simulink model "new_fusion_model"  (R2026a)
settings: Solver=VariableStepAuto  StopTime=180
InitFcn:
  | initNoise
  | initUKF
  | initKF
model workspace (MAT data in the model file):
  Ts = 0.05
undefined symbols (not defined in the file): Discrete, r_range, r_th_ac, r_th_ir, r_th_radar, Rkf, seed_ac, seed_ir, seed_radar_bearing, seed_radar_range, Time, x0kf
libraries: sharedTrackingLibrary x3, ctrlSharedLib x1

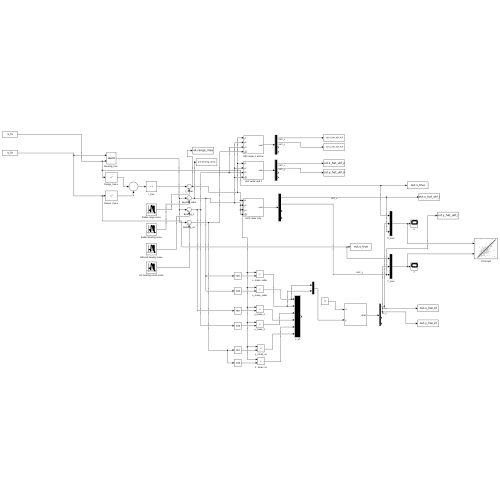
[thumbnail: Simulink's stored preview of the top-level diagram]
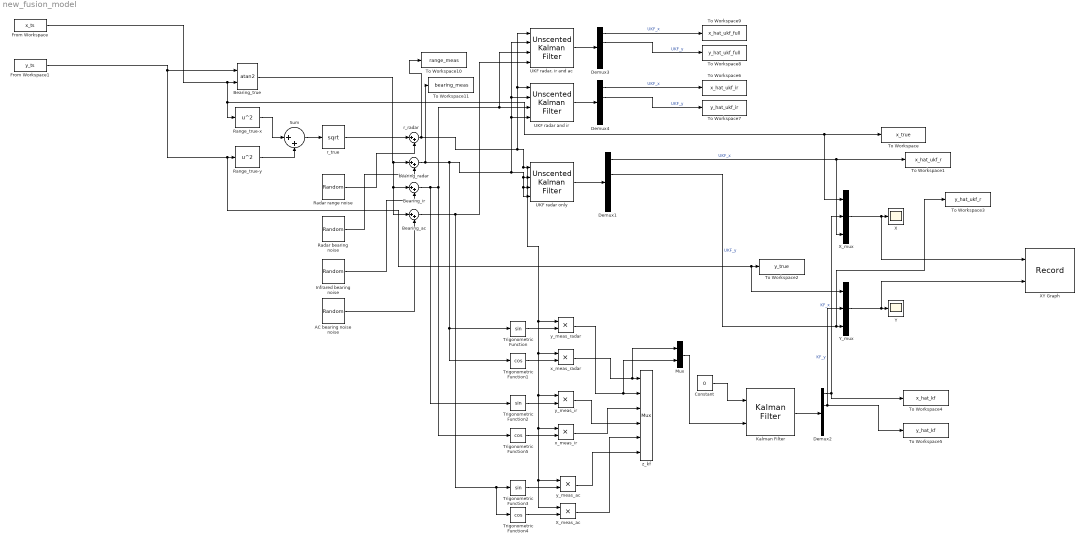
== system new_fusion_model ==
  AC bearing noise noise : RandomNumber  Variance=r_th_ac  Seed=seed_ac  SampleTime=4*Ts
  Bearing_ac : Sum  Inputs=|++
  Bearing_ir : Sum  Inputs=|++
  "Bearing_true " : Trigonometry  Operator=atan2
  Constant : Constant  Value=0
  Demux{1..4} (4 alike) : Demux
  From Workspace : FromWorkspace  VariableName=x_ts  SampleTime=Ts
  From Workspace1 : FromWorkspace  VariableName=y_ts  SampleTime=Ts
  Infrared bearing noise : RandomNumber  Variance=r_th_ir  Seed=seed_ir  SampleTime=2*Ts
  Kalman Filter : ctrlSharedLib/Kalman Filter  TimeDomain=Discrete-Time  UseCurrentEstimator=on  ModelSource=LTI State-Space Variable  ModelSourceVariable=sysKF  A=0.95  B=1  C=1  D=0  NumberOfStates=1  NumberOfInputs=1  NumberOfOutputs=1  Ts=-1  InitialEstimateSource=Dialog  X0=x0kf  P0=10  UseK=off  UseGH=off  G=1  TimeInvariantG=on  H=0  TimeInvariantH=on  NumberOfProcessNoiseInputs=1  Q=Qkf  TimeInvariantQ=on  R=Rkf  TimeInvariantR=on  N=0  TimeInvariantN=on  AddInputPort=on  AddEnablePort=off  OutputEstimatedY=off  OutputP=off
  Mux : Mux  Inputs=2
  Radar bearing noise : RandomNumber  Variance=r_th_radar  Seed=seed_radar_bearing  SampleTime=Ts
  Radar range noise : RandomNumber  Variance=r_range  Seed=seed_radar_range  SampleTime=Ts
  Range_true-x : Math  Operator=square
  Range_true-y : Math  Operator=square
  Sum : Sum  Inputs=|++
  To Workspace : ToWorkspace  VariableName=x_true  SaveFormat=Timeseries  SampleTime=Ts
  To Workspace1 : ToWorkspace  VariableName=x_hat_ukf_r  SaveFormat=Timeseries  SampleTime=Ts
  To Workspace10 : ToWorkspace  VariableName=range_meas  SaveFormat=Timeseries  SampleTime=Ts
  To Workspace11 : ToWorkspace  VariableName=bearing_meas  SaveFormat=Timeseries  SampleTime=Ts
  To Workspace2 : ToWorkspace  VariableName=y_true  SaveFormat=Timeseries  SampleTime=Ts
  To Workspace3 : ToWorkspace  VariableName=y_hat_ukf_r  SaveFormat=Timeseries  SampleTime=Ts
  To Workspace4 : ToWorkspace  VariableName=x_hat_kf  SaveFormat=Timeseries  SampleTime=Ts
  To Workspace5 : ToWorkspace  VariableName=y_hat_kf  SaveFormat=Timeseries  SampleTime=Ts
  To Workspace6 : ToWorkspace  VariableName=x_hat_ukf_ir  SaveFormat=Timeseries  SampleTime=Ts
  To Workspace7 : ToWorkspace  VariableName=y_hat_ukf_ir  SaveFormat=Timeseries  SampleTime=Ts
  To Workspace8 : ToWorkspace  VariableName=y_hat_ukf_full  SaveFormat=Timeseries  SampleTime=Ts
  To Workspace9 : ToWorkspace  VariableName=x_hat_ukf_full  SaveFormat=Timeseries  SampleTime=Ts
  Trigonometric Function : Trigonometry
  Trigonometric Function1 : Trigonometry  Operator=cos
  Trigonometric Function2 : Trigonometry
  Trigonometric Function3 : Trigonometry
  Trigonometric Function4 : Trigonometry  Operator=cos
  Trigonometric Function5 : Trigonometry  Operator=cos
  UKF radar and ir : sharedTrackingLibrary/Unscented Kalman Filter  StateTransitionFcn=ukf_state_transition_2026  HasAdditiveProcessNoise=Additive  ProcessNoise=Q  HasTimeVaryingProcessNoise=off  HasStateTransitionFcnExtraArgument=0  InitialState=x0  InitialStateCovariance=P0  Alpha=1e-3  Beta=2  Kappa=0  MeasurementFcn1=ukf_radar_range_2026  HasMeasurementEnablePort1=off  HasAdditiveMeasurementNoise1=Additive  MeasurementNoise1=r_range  HasTimeVaryingMeasurementNoise1=off  HasMeasurementFcnExtraArgument1=0  HasMeasurementWrapping1=off  MeasurementFcn2=ukf_radar_bearing_2026  HasMeasurementEnablePort2=off  HasAdditiveMeasurementNoise2=Additive  MeasurementNoise2=r_th_radar  HasTimeVaryingMeasurementNoise2=off  HasMeasurementFcnExtraArgument2=0  HasMeasurementWrapping2=on  MeasurementFcn3=ukf_ir_bearing_2026  HasMeasurementEnablePort3=off  HasAdditiveMeasurementNoise3=Additive  MeasurementNoise3=r_th_ir  HasTimeVaryingMeasurementNoise3=off  HasMeasurementFcnExtraArgument3=0  HasMeasurementWrapping3=on  MeasurementFcn4=ukf_ac_bearing_2026  HasMeasurementEnablePort4=off  HasAdditiveMeasurementNoise4=Additive  MeasurementNoise4=r_th_ac  HasTimeVaryingMeasurementNoise4=off  HasMeasurementFcnExtraArgument4=0  HasMeasurementWrapping4=on  MeasurementFcn5=myMeasurementFcn  HasMeasurementEnablePort5=off  HasAdditiveMeasurementNoise5=Additive  MeasurementNoise5=1  HasTimeVaryingMeasurementNoise5=off  HasMeasurementFcnExtraArgument5=0  HasMeasurementWrapping5=off  EnableMultirate=off  StateTransitionFcnSampleTime=1  MeasurementFcn1SampleTime=1  MeasurementFcn2SampleTime=1  MeasurementFcn3SampleTime=1  MeasurementFcn4SampleTime=1  MeasurementFcn5SampleTime=1  UseCurrentEstimator=on  OutputStateCovariance=off  DataType=double  SampleTime=Ts  NumberOfMeasurements=4
      settings: LibrarySourceBlock=cstblocks/State Estimation/Unscented Kalman Filter
  UKF radar only : sharedTrackingLibrary/Unscented Kalman Filter  StateTransitionFcn=ukf_state_transition_2026  HasAdditiveProcessNoise=Additive  ProcessNoise=Q  HasTimeVaryingProcessNoise=off  HasStateTransitionFcnExtraArgument=0  InitialState=x0  InitialStateCovariance=P0  Alpha=1e-3  Beta=2  Kappa=0  MeasurementFcn1=ukf_radar_range_2026  HasMeasurementEnablePort1=off  HasAdditiveMeasurementNoise1=Additive  MeasurementNoise1=r_range  HasTimeVaryingMeasurementNoise1=off  HasMeasurementFcnExtraArgument1=0  HasMeasurementWrapping1=off  MeasurementFcn2=ukf_radar_bearing_2026  HasMeasurementEnablePort2=off  HasAdditiveMeasurementNoise2=Additive  MeasurementNoise2=r_th_radar  HasTimeVaryingMeasurementNoise2=off  HasMeasurementFcnExtraArgument2=0  HasMeasurementWrapping2=on  MeasurementFcn3=ukf_ir_bearing_2026  HasMeasurementEnablePort3=off  HasAdditiveMeasurementNoise3=Additive  MeasurementNoise3=r_th_ir  HasTimeVaryingMeasurementNoise3=off  HasMeasurementFcnExtraArgument3=0  HasMeasurementWrapping3=on  MeasurementFcn4=ukf_ac_bearing_2026  HasMeasurementEnablePort4=off  HasAdditiveMeasurementNoise4=Additive  MeasurementNoise4=r_th_ac  HasTimeVaryingMeasurementNoise4=off  HasMeasurementFcnExtraArgument4=0  HasMeasurementWrapping4=on  MeasurementFcn5=myMeasurementFcn  HasMeasurementEnablePort5=off  HasAdditiveMeasurementNoise5=Additive  MeasurementNoise5=1  HasTimeVaryingMeasurementNoise5=off  HasMeasurementFcnExtraArgument5=0  HasMeasurementWrapping5=off  EnableMultirate=off  StateTransitionFcnSampleTime=1  MeasurementFcn1SampleTime=1  MeasurementFcn2SampleTime=1  MeasurementFcn3SampleTime=1  MeasurementFcn4SampleTime=1  MeasurementFcn5SampleTime=1  UseCurrentEstimator=on  OutputStateCovariance=off  DataType=double  SampleTime=Ts  NumberOfMeasurements=4
      settings: LibrarySourceBlock=cstblocks/State Estimation/Unscented Kalman Filter
  "UKF radar, ir and ac" : sharedTrackingLibrary/Unscented Kalman Filter  StateTransitionFcn=ukf_state_transition_2026  HasAdditiveProcessNoise=Additive  ProcessNoise=Q  HasTimeVaryingProcessNoise=off  HasStateTransitionFcnExtraArgument=0  InitialState=x0  InitialStateCovariance=P0  Alpha=1e-3  Beta=2  Kappa=0  MeasurementFcn1=ukf_radar_range_2026  HasMeasurementEnablePort1=off  HasAdditiveMeasurementNoise1=Additive  MeasurementNoise1=r_range  HasTimeVaryingMeasurementNoise1=off  HasMeasurementFcnExtraArgument1=0  HasMeasurementWrapping1=off  MeasurementFcn2=ukf_radar_bearing_2026  HasMeasurementEnablePort2=off  HasAdditiveMeasurementNoise2=Additive  MeasurementNoise2=r_th_radar  HasTimeVaryingMeasurementNoise2=off  HasMeasurementFcnExtraArgument2=0  HasMeasurementWrapping2=on  MeasurementFcn3=ukf_ir_bearing_2026  HasMeasurementEnablePort3=off  HasAdditiveMeasurementNoise3=Additive  MeasurementNoise3=r_th_ir  HasTimeVaryingMeasurementNoise3=off  HasMeasurementFcnExtraArgument3=0  HasMeasurementWrapping3=on  MeasurementFcn4=ukf_ac_bearing_2026  HasMeasurementEnablePort4=off  HasAdditiveMeasurementNoise4=Additive  MeasurementNoise4=r_th_ac  HasTimeVaryingMeasurementNoise4=off  HasMeasurementFcnExtraArgument4=0  HasMeasurementWrapping4=on  MeasurementFcn5=myMeasurementFcn  HasMeasurementEnablePort5=off  HasAdditiveMeasurementNoise5=Additive  MeasurementNoise5=1  HasTimeVaryingMeasurementNoise5=off  HasMeasurementFcnExtraArgument5=0  HasMeasurementWrapping5=off  EnableMultirate=off  StateTransitionFcnSampleTime=1  MeasurementFcn1SampleTime=1  MeasurementFcn2SampleTime=1  MeasurementFcn3SampleTime=1  MeasurementFcn4SampleTime=1  MeasurementFcn5SampleTime=1  UseCurrentEstimator=on  OutputStateCovariance=off  DataType=double  SampleTime=Ts  NumberOfMeasurements=4
      settings: LibrarySourceBlock=cstblocks/State Estimation/Unscented Kalman Filter
  X : Scope
      settings: ActiveDisplayYMinimum=1197.71183530067  ActiveDisplayYMaximum=1993.9408738589041
  XY Graph : Record  NumPorts=2.0  FileSettingsInternal="{\"entries\":[{\"content\":{\"excelSettings\":{\"content\":{},\"type\":\"Streamout.ExcelSettings\"},\"parquetSettings\":{\"content\":{},\"type\":\"Streamout.ParquetSettings\"}},\"type\":\"Streamout.FileSettingStorage\",\"uuid\":\"\"}],\"packageUris\":[\"http:\\/\\/schema.mathworks.com\\/mf0\\/streamout_blocks\\/R2020a\"],\"version\":\"1.0\"}"  FrameSettings=[0, 0]  Layout=[1 1]  SignalsInternal="{\"entries\":[{\"content\":{\"signals\":[{\"content\":{\"blockPath\":[],\"dimensions\":[3],\"domain\":\"\",\"hasChildren\":true,\"lineColor\":\"#fe330a\",\"lineWidth\":2,\"port\":1,\"sid\":[\"\"],\"signalID\":1,\"signalName\":\"X_mux\"},\"type\":\"RecordBlkView.Signal\",\"uuid\":\"\"},{\"content\":{\"blockPath\":[],\"channel\":[1],\"dimensions\":[3],\"domain\":\"\",\"lineColor\":\"#22b573\",\"lineWidth\":2,\"parentID\":1,\"port\":1,\"sid\":[\"\"],\"signalID\":2,\"signalName\":\"X_mux\"},\"type\":\"RecordBlkView.Signal\",\"uuid\":\"\"},{\"content\":{\"blockPath\":[],\"dimensions\":[3],\"domain\":\"\",\"hasChildren\":true,\"lineColor\":\"#0072bd\",\"lineWidth\":2,\"port\":2,\"sid\":[\"\"],\"signalID\":3,\"signalName\":\"Y_mux\"},\"type\":\"RecordBlkView.Signal\",\"uuid\":\"\"},{\"content\":{\"blockPath\":[],\"channel\":[1],\"dimensions\":[3],\"domain\":\"\",\"lineColor\":\"#d95319\",\"lineWidth\":2,\"parentID\":3,\"port\":2,\"sid\":[\"\"],\"signalID\":4,\"signalName\":\"Y_mux\"},\"type\":\"RecordBlkView.Signal\",\"uuid\":\"\"}]},\"type\":\"RecordBlkView.InputSignals\",\"uuid\":\"\"}],\"packageUris\":[\"http:\\/\\/schema.mathworks.com\\/mf0\\/streamout_blocks\\/R2020a\"],\"version\":\"1.0\"}"  VisualizationBindings="{\"xyplotplugin\":{\"info\":[{\"series\":[],\"subplotID\":1}]}}"  CompatibilityTag=XY
  X_meas_ac : Product
  X_mux : Mux  Inputs=3
  Y : Scope
      settings: ActiveDisplayYMinimum=-371.43892562544306  ActiveDisplayYMaximum=1085.8134789155749
  Y_mux : Mux  Inputs=3
  bearing_radar : Sum  Inputs=|++
  r_radar : Sum  Inputs=|++
  r_true : Sqrt
  x_meas_ir : Product
  x_meas_radar : Product
  y_meas_ac : Product
  y_meas_ir : Product
  y_meas_radar : Product
  z_kf : Mux  Inputs=6
  wires:
  Range_true-x/1 -> Sum/1
  Range_true-y/1 -> Sum/2
  Sum/1 -> r_true/1
  r_true/1 -> r_radar/1
  Radar range noise/1 -> r_radar/2
  "Bearing_true "/1 -> Bearing_ir/1, Bearing_ac/1, bearing_radar/1
  Radar bearing noise/1 -> bearing_radar/2
  Infrared bearing noise/1 -> Bearing_ir/2
  AC bearing noise noise/1 -> Bearing_ac/2
  r_radar/1 -> To Workspace10/1, y_meas_radar/1, x_meas_radar/1, y_meas_ir/1, x_meas_ir/1, y_meas_ac/1, X_meas_ac/1, UKF radar only/1, "UKF radar, ir and ac"/1, UKF radar and ir/1
  bearing_radar/1 -> To Workspace11/1, Trigonometric Function/1, Trigonometric Function1/1, UKF radar only/3, UKF radar only/4, UKF radar only/2, UKF radar and ir/4, UKF radar and ir/2, "UKF radar, ir and ac"/2
  Bearing_ir/1 -> Trigonometric Function2/1, UKF radar and ir/3, "UKF radar, ir and ac"/3, Trigonometric Function5/1
  Bearing_ac/1 -> "UKF radar, ir and ac"/4, Trigonometric Function3/1, Trigonometric Function4/1
  UKF radar only/1 -> Demux1/1
  Demux1/1 -> To Workspace1/1, X_mux/3  "UKF_x"
  Trigonometric Function/1 -> y_meas_radar/2
  Trigonometric Function2/1 -> y_meas_ir/2
  Trigonometric Function5/1 -> x_meas_ir/2
  Trigonometric Function1/1 -> x_meas_radar/2
  Trigonometric Function4/1 -> X_meas_ac/2
  Trigonometric Function3/1 -> y_meas_ac/2
  x_meas_radar/1 -> Mux/1, z_kf/1
  y_meas_radar/1 -> z_kf/2, Mux/2
  x_meas_ir/1 -> z_kf/3
  y_meas_ir/1 -> z_kf/4
  X_meas_ac/1 -> z_kf/5
  y_meas_ac/1 -> z_kf/6
  Constant/1 -> Kalman Filter/1
  Kalman Filter/1 -> Demux2/1
  Demux2/1 -> To Workspace4/1, X_mux/2  "KF_x"
  X_mux/1 -> XY Graph/1, X/1
  Demux1/2 -> To Workspace3/1, Y_mux/3  "UKF_y"
  Y_mux/1 -> XY Graph/2, Y/1
  Demux2/2 -> To Workspace5/1, Y_mux/2  "KF_y"
  Mux/1 -> Kalman Filter/2
  "UKF radar, ir and ac"/1 -> Demux3/1
  UKF radar and ir/1 -> Demux4/1
  Demux4/1 -> To Workspace6/1  "UKF_x"
  Demux4/2 -> To Workspace7/1  "UKF_y"
  Demux3/1 -> To Workspace9/1  "UKF_x"
  Demux3/2 -> To Workspace8/1  "UKF_y"
  From Workspace/1 -> Range_true-x/1, To Workspace/1, X_mux/1, "Bearing_true "/2
  From Workspace1/1 -> "Bearing_true "/1, Y_mux/1, To Workspace2/1, Range_true-y/1
